simulink model "ssc_auto_ev_20b"  (R2020b)
settings: Solver=VariableStepAuto  StartTime=0.0  StopTime=200  RelTol=1e-3  AbsTol=1e-3
PreLoadFcn:
  | % Simulation parameters
  | dt = 0.01;
  | 
  | % Battery cell parameters
  | ssc_lithium_cell_1RC_ini
  | Nseries = 100;
  | Nparallel = 10;
  | 
  | % Motor parameters
  | max_torque = 220;
  | max_power = 80e3;
  | 
  | % Vehicle parameters
  | vehicle_mass = 4000;
  | wheel_radius = 0.35;
  | area = 5;
  | drag_coefficient = 0.25;
  | air_density = 1.225;
  | gravity = 9.81;
  | rolling_res_ratio = 0.015;
  | 
  | % Differential drive parameters
  | gear_ratio = 12;
  | 
  | % Simplified braking system parameters
  | force_max_pedal = 500;
  | braking_torque_to_pedal_force_ratio = -16;
  | 
  | % Vehicle controller parameters
  | hill_hold_max_speed = 0.5;
  | 
  | % Water properties for cooling circuit
  | load WaterProperties
  | 
  | % Input signals for Signal Editor block
  | load ssc_auto_ev_Inputs
values from neighbouring files (symbols this model uses):
  C1_LUT = [1913.6 4625.7 23306 10736 18036 12251 9022.9 12447 18872 40764 18721 33630 ... (21 elements, 7x3)]    [ssc_auto_ev_param.mat]
  Capacity_LUT = [28.0081 27.625 27.6392]    [ssc_auto_ev_param.mat]
  cell_Cp_heat = 810.5328    [ssc_auto_ev_param.mat]
  cell_mass = 1    [ssc_auto_ev_param.mat]
  Em_LUT = [3.4966 3.5519 3.6183 3.7066 3.9131 4.0748 4.1923 3.5057 3.566 3.6337 3.7127 3.9259 ... (21 elements, 7x3)]    [ssc_auto_ev_param.mat]
  Qe_init = 15.6845    [ssc_auto_ev_param.mat]
  R0_LUT = [0.0117 0.011 0.0114 0.0107 0.0107 0.0113 0.0116 0.0085 0.0085 0.0087 0.0082 0.0083 ... (21 elements, 7x3)]    [ssc_auto_ev_param.mat]
  R1_LUT = [0.0109 0.0069 0.0047 0.0034 0.0033 0.0033 0.0028 0.0029 0.0024 0.0026 0.0016 0.0023 ... (21 elements, 7x3)]    [ssc_auto_ev_param.mat]
  SOC_LUT = [0 0.1 0.25 0.5 0.75 0.9 1]    [ssc_auto_ev_param.mat]
  T_init = 293.15    [ssc_auto_ev_param.mat]
  Temperature_LUT = [278.15 293.15 313.15]    [ssc_auto_ev_param.mat]
undefined symbols (not defined in the file or in its folder): DiscIntNeverNeededParam, K, Lambda, tau, x0
libraries: fl_lib x656, nesl_utility x86, simulink x21, LiBatteryElements_lib x16, SignalEditorBlockLib x4, simulink_extras x4
(part 10 of 13)

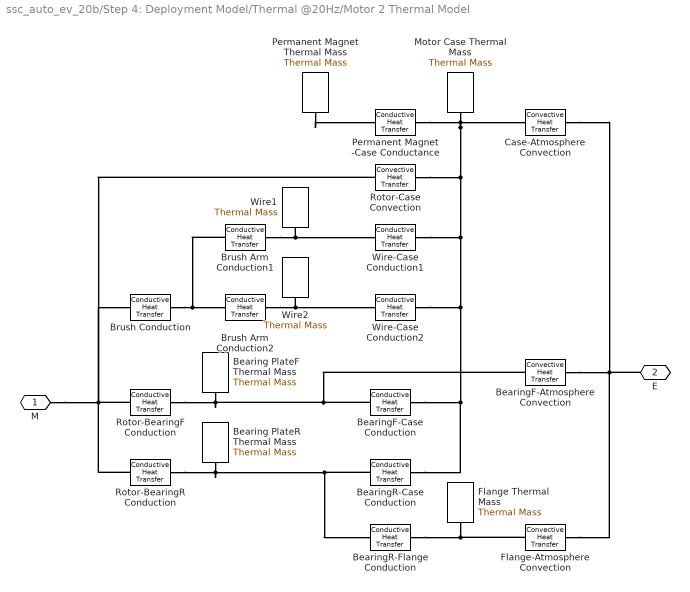
== system ssc_auto_ev_20b/Step 4: Deployment Model/Thermal @20Hz/Motor 2 Thermal Model ==
  Bearing PlateF Thermal Mass : fl_lib/Thermal/Thermal Elements/Thermal Mass  mass=0.6 kg  sp_heat=447 J/kg/K  T_specify=off  T_priority=High  T=300 K  T_nominal_specify=off  T_nominal_unit=K  T_nominal_value=1  Q_specify=off  Q_priority=None  Q=0 W  Q_nominal_specify=off  Q_nominal_unit=W  Q_nominal_value=1
      settings: SourceProductBaseCode=PW,SS,VE
  Bearing PlateR Thermal Mass : fl_lib/Thermal/Thermal Elements/Thermal Mass  mass=0.6 kg  sp_heat=447 J/kg/K  T_specify=off  T_priority=High  T=300 K  T_nominal_specify=off  T_nominal_unit=K  T_nominal_value=1  Q_specify=off  Q_priority=None  Q=0 W  Q_nominal_specify=off  Q_nominal_unit=W  Q_nominal_value=1
      settings: SourceProductBaseCode=PW,SS,VE
  BearingF-Atmosphere Convection : fl_lib/Thermal/Thermal Elements/Convective Heat Transfer  area=274.6 cm^2  heat_tr_coeff=123.5 W/(m^2 * K)  T_specify=off  T_priority=None  T=0 K  T_nominal_specify=off  T_nominal_unit=K  T_nominal_value=1  Q_specify=off  Q_priority=None  Q=0 W  Q_nominal_specify=off  Q_nominal_unit=W  Q_nominal_value=1
      settings: SourceProductBaseCode=PW,SS,VE
  BearingF-Case Conduction : fl_lib/Thermal/Thermal Elements/Conductive Heat Transfer  area=145 cm^2  thickness=18 cm  th_cond=80.2 W/(m*K)  T_specify=off  T_priority=None  T=0 K  T_nominal_specify=off  T_nominal_unit=K  T_nominal_value=1  Q_specify=off  Q_priority=None  Q=0 W  Q_nominal_specify=off  Q_nominal_unit=W  Q_nominal_value=1
      settings: SourceProductBaseCode=PW,SS,VE
  BearingR-Case Conduction : fl_lib/Thermal/Thermal Elements/Conductive Heat Transfer  area=145 cm^2  thickness=25 cm  th_cond=80.2 W/(m*K)  T_specify=off  T_priority=None  T=0 K  T_nominal_specify=off  T_nominal_unit=K  T_nominal_value=1  Q_specify=off  Q_priority=None  Q=0 W  Q_nominal_specify=off  Q_nominal_unit=W  Q_nominal_value=1
      settings: SourceProductBaseCode=PW,SS,VE
  BearingR-Flange Conduction : fl_lib/Thermal/Thermal Elements/Conductive Heat Transfer  area=34.5 cm^2  thickness=14 cm  th_cond=80.2 W/(m*K)  T_specify=off  T_priority=None  T=0 K  T_nominal_specify=off  T_nominal_unit=K  T_nominal_value=1  Q_specify=off  Q_priority=None  Q=0 W  Q_nominal_specify=off  Q_nominal_unit=W  Q_nominal_value=1
      settings: SourceProductBaseCode=PW,SS,VE
  Brush Conduction : fl_lib/Thermal/Thermal Elements/Conductive Heat Transfer  area=3*5 cm^2  thickness=4 cm  th_cond=1.7 W/(m*K)  T_specify=off  T_priority=None  T=0 K  T_nominal_specify=off  T_nominal_unit=K  T_nominal_value=1  Q_specify=off  Q_priority=None  Q=0 W  Q_nominal_specify=off  Q_nominal_unit=W  Q_nominal_value=1
      settings: SourceProductBaseCode=PW,SS,VE
  Brush Arm Conduction1 : fl_lib/Thermal/Thermal Elements/Conductive Heat Transfer  area=3*5 cm^2  thickness=4 cm  th_cond=1.7 W/(m*K)  T_specify=off  T_priority=None  T=0 K  T_nominal_specify=off  T_nominal_unit=K  T_nominal_value=1  Q_specify=off  Q_priority=None  Q=0 W  Q_nominal_specify=off  Q_nominal_unit=W  Q_nominal_value=1
      settings: SourceProductBaseCode=PW,SS,VE
  Brush Arm Conduction2 : fl_lib/Thermal/Thermal Elements/Conductive Heat Transfer  area=3*5 cm^2  thickness=4 cm  th_cond=1.7 W/(m*K)  T_specify=off  T_priority=None  T=0 K  T_nominal_specify=off  T_nominal_unit=K  T_nominal_value=1  Q_specify=off  Q_priority=None  Q=0 W  Q_nominal_specify=off  Q_nominal_unit=W  Q_nominal_value=1
      settings: SourceProductBaseCode=PW,SS,VE
  Case-Atmosphere Convection : fl_lib/Thermal/Thermal Elements/Convective Heat Transfer  area=4240 cm^2  heat_tr_coeff=26.8 W/(m^2 * K)  T_specify=off  T_priority=None  T=0 K  T_nominal_specify=off  T_nominal_unit=K  T_nominal_value=1  Q_specify=off  Q_priority=None  Q=0 W  Q_nominal_specify=off  Q_nominal_unit=W  Q_nominal_value=1
      settings: SourceProductBaseCode=PW,SS,VE
  Flange Thermal Mass : fl_lib/Thermal/Thermal Elements/Thermal Mass  mass=1.6 kg  sp_heat=447 J/kg/K  T_specify=off  T_priority=High  T=300 K  T_nominal_specify=off  T_nominal_unit=K  T_nominal_value=1  Q_specify=off  Q_priority=None  Q=0 W  Q_nominal_specify=off  Q_nominal_unit=W  Q_nominal_value=1
      settings: SourceProductBaseCode=PW,SS,VE
  Flange-Atmosphere Convection : fl_lib/Thermal/Thermal Elements/Convective Heat Transfer  area=324 cm^2  heat_tr_coeff=123.4 W/(m^2 * K)  T_specify=off  T_priority=None  T=0 K  T_nominal_specify=off  T_nominal_unit=K  T_nominal_value=1  Q_specify=off  Q_priority=None  Q=0 W  Q_nominal_specify=off  Q_nominal_unit=W  Q_nominal_value=1
      settings: SourceProductBaseCode=PW,SS,VE
  Motor Case Thermal Mass : fl_lib/Thermal/Thermal Elements/Thermal Mass  mass=3.8 kg  sp_heat=903 J/kg/K  T_specify=off  T_priority=High  T=300 K  T_nominal_specify=off  T_nominal_unit=K  T_nominal_value=1  Q_specify=off  Q_priority=None  Q=0 W  Q_nominal_specify=off  Q_nominal_unit=W  Q_nominal_value=1
      settings: SourceProductBaseCode=PW,SS,VE
  Permanent Magnet Thermal Mass : fl_lib/Thermal/Thermal Elements/Thermal Mass  mass=3.6 kg  sp_heat=447 J/kg/K  T_specify=off  T_priority=High  T=300 K  T_nominal_specify=off  T_nominal_unit=K  T_nominal_value=1  Q_specify=off  Q_priority=None  Q=0 W  Q_nominal_specify=off  Q_nominal_unit=W  Q_nominal_value=1
      settings: SourceProductBaseCode=PW,SS,VE
  Permanent Magnet -Case Conductance : fl_lib/Thermal/Thermal Elements/Conductive Heat Transfer  area=4350 cm^2  thickness=26 cm  th_cond=80.2 W/(m*K)  T_specify=off  T_priority=None  T=0 K  T_nominal_specify=off  T_nominal_unit=K  T_nominal_value=1  Q_specify=off  Q_priority=None  Q=0 W  Q_nominal_specify=off  Q_nominal_unit=W  Q_nominal_value=1
      settings: SourceProductBaseCode=PW,SS,VE
  Rotor-BearingF Conduction : fl_lib/Thermal/Thermal Elements/Conductive Heat Transfer  area=26.4 cm^2  thickness=2.5 cm  th_cond=80.2 W/(m*K)  T_specify=off  T_priority=None  T=0 K  T_nominal_specify=off  T_nominal_unit=K  T_nominal_value=1  Q_specify=off  Q_priority=None  Q=0 W  Q_nominal_specify=off  Q_nominal_unit=W  Q_nominal_value=1
      settings: SourceProductBaseCode=PW,SS,VE
  Rotor-BearingR Conduction : fl_lib/Thermal/Thermal Elements/Conductive Heat Transfer  area=26.4 cm^2  thickness=2.5 cm  th_cond=80.2 W/(m*K)  T_specify=off  T_priority=None  T=0 K  T_nominal_specify=off  T_nominal_unit=K  T_nominal_value=1  Q_specify=off  Q_priority=None  Q=0 W  Q_nominal_specify=off  Q_nominal_unit=W  Q_nominal_value=1
      settings: SourceProductBaseCode=PW,SS,VE
  Rotor-Case Convection : fl_lib/Thermal/Thermal Elements/Convective Heat Transfer  area=1240 cm^2  heat_tr_coeff=210 W/(m^2 * K)  T_specify=off  T_priority=None  T=0 K  T_nominal_specify=off  T_nominal_unit=K  T_nominal_value=1  Q_specify=off  Q_priority=None  Q=0 W  Q_nominal_specify=off  Q_nominal_unit=W  Q_nominal_value=1
      settings: SourceProductBaseCode=PW,SS,VE
  Wire-Case Conduction1 : fl_lib/Thermal/Thermal Elements/Conductive Heat Transfer  area=1 cm^2  thickness=0.2 cm  th_cond=4 W/(m*K)  T_specify=off  T_priority=None  T=0 K  T_nominal_specify=off  T_nominal_unit=K  T_nominal_value=1  Q_specify=off  Q_priority=None  Q=0 W  Q_nominal_specify=off  Q_nominal_unit=W  Q_nominal_value=1
      settings: SourceProductBaseCode=PW,SS,VE
  Wire-Case Conduction2 : fl_lib/Thermal/Thermal Elements/Conductive Heat Transfer  area=1 cm^2  thickness=0.2 cm  th_cond=4 W/(m*K)  T_specify=off  T_priority=None  T=0 K  T_nominal_specify=off  T_nominal_unit=K  T_nominal_value=1  Q_specify=off  Q_priority=None  Q=0 W  Q_nominal_specify=off  Q_nominal_unit=W  Q_nominal_value=1
      settings: SourceProductBaseCode=PW,SS,VE
  Wire1 : fl_lib/Thermal/Thermal Elements/Thermal Mass  mass=0.05 kg  sp_heat=385 J/kg/K  T_specify=off  T_priority=High  T=300 K  T_nominal_specify=off  T_nominal_unit=K  T_nominal_value=1  Q_specify=off  Q_priority=None  Q=0 W  Q_nominal_specify=off  Q_nominal_unit=W  Q_nominal_value=1
      settings: SourceProductBaseCode=PW,SS,VE
  Wire2 : fl_lib/Thermal/Thermal Elements/Thermal Mass  mass=0.05 kg  sp_heat=385 J/kg/K  T_specify=off  T_priority=High  T=300 K  T_nominal_specify=off  T_nominal_unit=K  T_nominal_value=1  Q_specify=off  Q_priority=None  Q=0 W  Q_nominal_specify=off  Q_nominal_unit=W  Q_nominal_value=1
      settings: SourceProductBaseCode=PW,SS,VE
  M : PMIOPort  Side=Right
  E : PMIOPort  Port=2  Side=Left
  connections:
  Flange-Atmosphere Convection/RConn1 -- E/RConn1 -- BearingF-Atmosphere Convection/RConn1 -- Case-Atmosphere Convection/RConn1
  Motor Case Thermal Mass/LConn1 -- Case-Atmosphere Convection/LConn1 -- Permanent Magnet -Case Conductance/RConn1 -- Wire-Case Conduction1/RConn1 -- Wire-Case Conduction2/RConn1 -- BearingF-Case Conduction/RConn1 -- BearingR-Case Conduction/RConn1 -- Rotor-Case Convection/RConn1
  Rotor-BearingR Conduction/RConn1 -- Bearing PlateR Thermal Mass/LConn1 -- BearingR-Flange Conduction/LConn1 -- BearingR-Case Conduction/LConn1
  Flange-Atmosphere Convection/LConn1 -- BearingR-Flange Conduction/RConn1 -- Flange Thermal Mass/LConn1
  BearingF-Case Conduction/LConn1 -- BearingF-Atmosphere Convection/LConn1 -- Rotor-BearingF Conduction/RConn1 -- Bearing PlateF Thermal Mass/LConn1
  M/RConn1 -- Rotor-Case Convection/LConn1 -- Brush Conduction/LConn1 -- Rotor-BearingR Conduction/LConn1 -- Rotor-BearingF Conduction/LConn1
  Permanent Magnet Thermal Mass/LConn1 -- Permanent Magnet -Case Conductance/LConn1
  Brush Conduction/RConn1 -- Brush Arm Conduction1/LConn1 -- Brush Arm Conduction2/LConn1
  Brush Arm Conduction1/RConn1 -- Wire-Case Conduction1/LConn1 -- Wire1/LConn1
  Brush Arm Conduction2/RConn1 -- Wire-Case Conduction2/LConn1 -- Wire2/LConn1

== system ssc_auto_ev_20b/Step 4: Deployment Model/Thermal @20Hz/Port 2 Interface ==
  temperature : Inport
  Controlled Temperature Source : fl_lib/Thermal/Thermal Sources/Controlled Temperature Source
      settings: SourceProductBaseCode=PW,SS,VE
  Heat Flow Rate Sensor : fl_lib/Thermal/Thermal Sensors/Heat Flow Rate Sensor
      settings: SourceProductBaseCode=PW,SS,VE
  T2 : nesl_utility/Simulink-PS Converter  PhysicalDomain=network_engine_domain  SubClassName=ps_input  LeftPortType=input  RightPortType=output  PseudoPeriodic=off  Frequencies=[]  NoiseDistribution=none  NoiseParameters=[]  Unit=K  AffineConversion=off  FilteringAndDerivatives=provide  SimscapeFilterOrder=1  InputFilterTimeConstant=0.001  UdotUserProvided=0
      settings: SourceProductBaseCode=SS,PW,VE
  Thermal Reference : fl_lib/Thermal/Thermal Elements/Thermal Reference
      settings: SourceProductBaseCode=PW,SS,VE
  q2 : nesl_utility/PS-Simulink Converter  PhysicalDomain=network_engine_domain  SubClassName=ps_output  LeftPortType=input  RightPortType=output  PseudoPeriodic=off  Frequencies=[]  Unit=W  AffineConversion=off
      settings: SourceProductBaseCode=SS,PW,VE
  2 : PMIOPort  Side=Right
  heat flow : Outport
  wires:
  q2/1 -> heat flow/1
  temperature/1 -> T2/1
  connections:
  Heat Flow Rate Sensor/RConn2 -- Controlled Temperature Source/LConn1
  Thermal Reference/LConn1 -- Controlled Temperature Source/RConn2
  Heat Flow Rate Sensor/LConn1 -- 2/RConn1
  T2/RConn1 -- Controlled Temperature Source/RConn1
  q2/LConn1 -- Heat Flow Rate Sensor/RConn1

== system ssc_auto_ev_20b/Step 4: Deployment Model/Thermal @20Hz/Port 2 Interface1 ==
  temperature : Inport
  Controlled Temperature Source : fl_lib/Thermal/Thermal Sources/Controlled Temperature Source
      settings: SourceProductBaseCode=PW,SS,VE
  Heat Flow Rate Sensor : fl_lib/Thermal/Thermal Sensors/Heat Flow Rate Sensor
      settings: SourceProductBaseCode=PW,SS,VE
  T2 : nesl_utility/Simulink-PS Converter  PhysicalDomain=network_engine_domain  SubClassName=ps_input  LeftPortType=input  RightPortType=output  PseudoPeriodic=off  Frequencies=[]  NoiseDistribution=none  NoiseParameters=[]  Unit=K  AffineConversion=off  FilteringAndDerivatives=provide  SimscapeFilterOrder=1  InputFilterTimeConstant=0.001  UdotUserProvided=0
      settings: SourceProductBaseCode=SS,PW,VE
  Thermal Reference : fl_lib/Thermal/Thermal Elements/Thermal Reference
      settings: SourceProductBaseCode=PW,SS,VE
  q2 : nesl_utility/PS-Simulink Converter  PhysicalDomain=network_engine_domain  SubClassName=ps_output  LeftPortType=input  RightPortType=output  PseudoPeriodic=off  Frequencies=[]  Unit=W  AffineConversion=off
      settings: SourceProductBaseCode=SS,PW,VE
  2 : PMIOPort  Side=Right
  heat flow : Outport
  wires:
  q2/1 -> heat flow/1
  temperature/1 -> T2/1
  connections:
  Heat Flow Rate Sensor/RConn2 -- Controlled Temperature Source/LConn1
  Thermal Reference/LConn1 -- Controlled Temperature Source/RConn2
  Heat Flow Rate Sensor/LConn1 -- 2/RConn1
  T2/RConn1 -- Controlled Temperature Source/RConn1
  q2/LConn1 -- Heat Flow Rate Sensor/RConn1

== system ssc_auto_ev_20b/Step 4: Deployment Model/Thermal @20Hz/Port 2 Interface2 ==
  temperature : Inport
  Controlled Temperature Source : fl_lib/Thermal/Thermal Sources/Controlled Temperature Source
      settings: SourceProductBaseCode=PW,SS,VE
  Heat Flow Rate Sensor : fl_lib/Thermal/Thermal Sensors/Heat Flow Rate Sensor
      settings: SourceProductBaseCode=PW,SS,VE
  T2 : nesl_utility/Simulink-PS Converter  PhysicalDomain=network_engine_domain  SubClassName=ps_input  LeftPortType=input  RightPortType=output  PseudoPeriodic=off  Frequencies=[]  NoiseDistribution=none  NoiseParameters=[]  Unit=K  AffineConversion=off  FilteringAndDerivatives=provide  SimscapeFilterOrder=1  InputFilterTimeConstant=0.001  UdotUserProvided=0
      settings: SourceProductBaseCode=SS,PW,VE
  Thermal Reference : fl_lib/Thermal/Thermal Elements/Thermal Reference
      settings: SourceProductBaseCode=PW,SS,VE
  q2 : nesl_utility/PS-Simulink Converter  PhysicalDomain=network_engine_domain  SubClassName=ps_output  LeftPortType=input  RightPortType=output  PseudoPeriodic=off  Frequencies=[]  Unit=W  AffineConversion=off
      settings: SourceProductBaseCode=SS,PW,VE
  2 : PMIOPort  Side=Right
  heat flow : Outport
  wires:
  temperature/1 -> T2/1
  q2/1 -> heat flow/1
  connections:
  q2/LConn1 -- Heat Flow Rate Sensor/RConn1
  T2/RConn1 -- Controlled Temperature Source/RConn1
  Heat Flow Rate Sensor/LConn1 -- 2/RConn1
  Thermal Reference/LConn1 -- Controlled Temperature Source/RConn2
  Heat Flow Rate Sensor/RConn2 -- Controlled Temperature Source/LConn1

== system ssc_auto_ev_20b/Step 4: Deployment Model/Vehicle and drive @100Hz/Motor Drive ==
  iRef : Inport
  DC Motor1 : Subsystem  Tag=PublishSubsystem
      mask Display:
      | % Circle, in/out, and 'M'
      | image('ssc_dcmotor_maskicon.png');
      | 
      | % % Circle
      | % plot(sin(0:0.1:2.2*pi)*0.9,cos(0:0.1:2.2*pi)*0.9);
      | %
      | % % In/out
      | % plot([-1.3 -0.9],[0 0]);
      | % plot([1.3 0.9],[0 0]);
      | %
      | % % 'M'
      | % plot([0.5 0.5],[-0.5 0.5]);
      | % plot([-0.5 -0.5],[-0.5 0.5]);
      | % plot([0.5 0],[0.5 -0.5]);
      | % plot([-0.5 0],[0.5 -0.5]);
      | 
      | % Plot points to set plot range
      | color('white');plot(1.5,1.5);plot(-1.5,-1.5)
      | color('black');
      | 
      | port_label('RConn',1,'R');
      | port_label('RConn',2,'C');
      | port_label('LConn',1,'V+');
      | port_label('LConn',2,'V-');
  DC Motor2 : Subsystem  Tag=PublishSubsystem
      mask Display:
      | % Circle, in/out, and 'M'
      | image('ssc_dcmotor_maskicon.png');
      | 
      | % % Circle
      | % plot(sin(0:0.1:2.2*pi)*0.9,cos(0:0.1:2.2*pi)*0.9);
      | %
      | % % In/out
      | % plot([-1.3 -0.9],[0 0]);
      | % plot([1.3 0.9],[0 0]);
      | %
      | % % 'M'
      | % plot([0.5 0.5],[-0.5 0.5]);
      | % plot([-0.5 -0.5],[-0.5 0.5]);
      | % plot([0.5 0],[0.5 -0.5]);
      | % plot([-0.5 0],[0.5 -0.5]);
      | 
      | % Plot points to set plot range
      | color('white');plot(1.5,1.5);plot(-1.5,-1.5)
      | color('black');
      | 
      | port_label('RConn',1,'R');
      | port_label('RConn',2,'C');
      | port_label('LConn',1,'V+');
      | port_label('LConn',2,'V-');
  Ideal Rotational Motion Sensor : fl_lib/Mechanical/Mechanical Sensors/Ideal Rotational Motion Sensor  wrap_angle=simscape.enum.onoff.off  offset=0 rad
      settings: SourceProductBaseCode=PW,SS,VE
  MRRef : fl_lib/Mechanical/Rotational Elements/Mechanical Rotational Reference
      settings: SourceProductBaseCode=PW,SS,VE
  MRRef1 : fl_lib/Mechanical/Rotational Elements/Mechanical Rotational Reference
      settings: SourceProductBaseCode=PW,SS,VE
  MRRef2 : fl_lib/Mechanical/Rotational Elements/Mechanical Rotational Reference
      settings: SourceProductBaseCode=PW,SS,VE
  Motor Torque Controller 1 (System-Level Representation) : Subsystem
      settings: PortSchema="{\"entries\":[{\"content\":{\"sides\":[{\"content\":{\"connectorIds\":[\"LConn1\",\"LConn2\"]},\"type\":\"ConnectorPlacement.EquallySpacedRectSide\",\"uuid\":\"fa610323-4e51-4b68-84d8-5520af174050\"},{\"content\":{\"connectorIds\":[\"RConn1\",\"RConn2\"],\"side\":\"RIGHT\"},\"type\":\"ConnectorPlacement.EquallySpacedRectSide\",\"uuid\":\"4363b90b-a4e0-4b49-9dec-cc6d130d9345\"},{\"content\":{\"connectorIds\":[\"LConn3\"],\"side\":\"TOP\"},\"type\":\"ConnectorPlacement.EquallySpacedRectSide\",\"uuid\":\"1b5285b6-bf42-4633-bccd-78a8c0464c36\"}]},\"type\":\"ConnectorPlacement.EquallySpacedConnector\",\"uuid\":\"5522e717-4ae9-420d-ac3d-a671d244aac1\"}],\"packageUris\":[\"http://schema.mathworks.com/mf0/Connector/R2020b\"],\"version\":\"1.0\"}"
  Motor Torque Controller 1 (System-Level Representation)1 : Subsystem
      settings: PortSchema="{\"entries\":[{\"content\":{\"sides\":[{\"content\":{\"connectorIds\":[\"LConn1\",\"LConn2\"]},\"type\":\"ConnectorPlacement.EquallySpacedRectSide\",\"uuid\":\"fa610323-4e51-4b68-84d8-5520af174050\"},{\"content\":{\"connectorIds\":[\"RConn1\",\"RConn2\"],\"side\":\"RIGHT\"},\"type\":\"ConnectorPlacement.EquallySpacedRectSide\",\"uuid\":\"4363b90b-a4e0-4b49-9dec-cc6d130d9345\"},{\"content\":{\"connectorIds\":[\"LConn3\"],\"side\":\"TOP\"},\"type\":\"ConnectorPlacement.EquallySpacedRectSide\",\"uuid\":\"1b5285b6-bf42-4633-bccd-78a8c0464c36\"}]},\"type\":\"ConnectorPlacement.EquallySpacedConnector\",\"uuid\":\"5522e717-4ae9-420d-ac3d-a671d244aac1\"}],\"packageUris\":[\"http://schema.mathworks.com/mf0/Connector/R2020b\"],\"version\":\"1.0\"}"
  Sensing wMotor : Subsystem
      mask Display: disp('w');
  Simulink-PS G1 : nesl_utility/Simulink-PS Converter  PhysicalDomain=network_engine_domain  SubClassName=ps_input  LeftPortType=input  RightPortType=output  PseudoPeriodic=off  Frequencies=[]  NoiseDistribution=none  NoiseParameters=[]  Unit=A  AffineConversion=off  FilteringAndDerivatives=zero  SimscapeFilterOrder=1  InputFilterTimeConstant=1e-6  UdotUserProvided=1
      settings: SourceProductBaseCode=SS,PW,VE
  Winding-Iron Conductance/1 : fl_lib/Thermal/Thermal Elements/Conductive Heat Transfer  area=250 cm^2  thickness=0.2 cm  th_cond=360 W/(m*K)  T_specify=off  T_priority=None  T=0 K  T_nominal_specify=off  T_nominal_unit=K  T_nominal_value=1  Q_specify=off  Q_priority=None  Q=0 W  Q_nominal_specify=off  Q_nominal_unit=W  Q_nominal_value=1
      settings: SourceProductBaseCode=PW,SS,VE
  Winding-Iron Conductance/2 : fl_lib/Thermal/Thermal Elements/Conductive Heat Transfer  area=250 cm^2  thickness=0.2 cm  th_cond=360 W/(m*K)  T_specify=off  T_priority=None  T=0 K  T_nominal_specify=off  T_nominal_unit=K  T_nominal_value=1  Q_specify=off  Q_priority=None  Q=0 W  Q_nominal_specify=off  Q_nominal_unit=W  Q_nominal_value=1
      settings: SourceProductBaseCode=PW,SS,VE
  + : PMIOPort  Side=Left
  - : PMIOPort  Port=2  Side=Left
  R : PMIOPort  Port=3  Side=Right
  M1 : PMIOPort  Port=4  Side=Left
  M2 : PMIOPort  Port=5  Side=Left
  w : Outport  VectorParamsAs1DForOutWhenUnconnected=off
  wires:
  iRef/1 -> Simulink-PS G1/1
  Sensing wMotor/1(SL) -> w/1
  connections:
  M2/RConn1 -- Winding-Iron Conductance/2/LConn1
  M1/RConn1 -- Winding-Iron Conductance/1/LConn1
  Winding-Iron Conductance/2/RConn1 -- DC Motor2/LConn3
  Winding-Iron Conductance/1/RConn1 -- DC Motor1/LConn3
  DC Motor2/LConn2 -- Motor Torque Controller 1 (System-Level Representation)1/LConn2
  DC Motor2/LConn1 -- Motor Torque Controller 1 (System-Level Representation)1/LConn1
  DC Motor2/RConn2 -- MRRef2/LConn1
  Motor Torque Controller 1 (System-Level Representation)1/LConn3 -- Motor Torque Controller 1 (System-Level Representation)/LConn3 -- Simulink-PS G1/RConn1
  DC Motor1/LConn2 -- Motor Torque Controller 1 (System-Level Representation)/LConn2
  Motor Torque Controller 1 (System-Level Representation)/RConn2 -- Motor Torque Controller 1 (System-Level Representation)1/RConn2 -- -/RConn1
  Motor Torque Controller 1 (System-Level Representation)/RConn1 -- Motor Torque Controller 1 (System-Level Representation)1/RConn1 -- +/RConn1
  Motor Torque Controller 1 (System-Level Representation)/LConn1 -- DC Motor1/LConn1
  MRRef1/LConn1 -- Ideal Rotational Motion Sensor/RConn1
  DC Motor1/RConn2 -- MRRef/LConn1
  R/RConn1 -- Ideal Rotational Motion Sensor/LConn1 -- DC Motor2/RConn1 -- DC Motor1/RConn1
  Ideal Rotational Motion Sensor/RConn2 -- Sensing wMotor/LConn1

== system ssc_auto_ev_20b/Step 4: Deployment Model/Vehicle and drive @100Hz/Port 1 Interface1 ==
  heat flow : Inport
  Controlled Temperature Source : fl_lib/Thermal/Thermal Sources/Controlled Temperature Source
      settings: SourceProductBaseCode=PW,SS,VE
  Heat Flow Rate Sensor : fl_lib/Thermal/Thermal Sensors/Heat Flow Rate Sensor
      settings: SourceProductBaseCode=PW,SS,VE
  Interface : Subsystem  Variant=on  VariantControlMode=label  VariantControl=Variant1  LabelModeActiveChoice=Discrete
      settings: PortSchema="{\"entries\":[{\"content\":{\"sides\":[{\"content\":{\"connectorIds\":[\"In1\",\"Out2\"]},\"type\":\"ConnectorPlacement.EquallySpacedRectSide\",\"uuid\":\"aa56821c-7799-44e3-b228-553c5b43a68d\"},{\"content\":{\"connectorIds\":[\"In2\",\"Out1\"],\"side\":\"RIGHT\"},\"type\":\"ConnectorPlacement.EquallySpacedRectSide\",\"uuid\":\"8658dee5-55e2-4f33-bdec-e6600ce27fc1\"},{\"content\":{\"connectorIds\":[],\"side\":\"TOP\"},\"type\":\"ConnectorPlacement.EquallySpacedRectSide\",\"uuid\":\"2effe9c6-8e61-4f0c-a39b-329d9ffc707d\"}]},\"type\":\"ConnectorPlacement.EquallySpacedConnector\",\"uuid\":\"c8fc8444-dfc7-49a5-9550-b957635f7d8f\"}],\"packageUris\":[\"http://schema.mathworks.com/mf0/Connector/R2020b\"],\"version\":\"1.0\"}"
  T1 : nesl_utility/Simulink-PS Converter  PhysicalDomain=network_engine_domain  SubClassName=ps_input  LeftPortType=input  RightPortType=output  PseudoPeriodic=off  Frequencies=[]  NoiseDistribution=none  NoiseParameters=[]  Unit=K  AffineConversion=off  FilteringAndDerivatives=provide  SimscapeFilterOrder=1  InputFilterTimeConstant=0.001  UdotUserProvided=0
      settings: SourceProductBaseCode=SS,PW,VE
  Thermal Reference : fl_lib/Thermal/Thermal Elements/Thermal Reference
      settings: SourceProductBaseCode=PW,SS,VE
  q1 : nesl_utility/PS-Simulink Converter  PhysicalDomain=network_engine_domain  SubClassName=ps_output  LeftPortType=input  RightPortType=output  PseudoPeriodic=off  Frequencies=[]  Unit=W  AffineConversion=off
      settings: SourceProductBaseCode=SS,PW,VE
  1 : PMIOPort  Side=Left
  temperature : Outport
  wires:
  Interface/1(across2) -> temperature/1
  q1/1 -> Interface/1(through1)
  heat flow/1 -> Interface/2(through2)
  Interface/2(across1) -> T1/1
  connections:
  Heat Flow Rate Sensor/RConn2 -- Controlled Temperature Source/LConn1
  Heat Flow Rate Sensor/LConn1 -- 1/RConn1
  q1/LConn1 -- Heat Flow Rate Sensor/RConn1
  Thermal Reference/LConn1 -- Controlled Temperature Source/RConn2
  Controlled Temperature Source/RConn1 -- T1/RConn1

== system ssc_auto_ev_20b/Step 4: Deployment Model/Vehicle and drive @100Hz/Port 1 Interface2 ==
  heat flow : Inport
  Controlled Temperature Source : fl_lib/Thermal/Thermal Sources/Controlled Temperature Source
      settings: SourceProductBaseCode=PW,SS,VE
  Heat Flow Rate Sensor : fl_lib/Thermal/Thermal Sensors/Heat Flow Rate Sensor
      settings: SourceProductBaseCode=PW,SS,VE
  Interface : Subsystem  Variant=on  VariantControlMode=label  VariantControl=Variant1  LabelModeActiveChoice=Discrete
      settings: PortSchema="{\"entries\":[{\"content\":{\"sides\":[{\"content\":{\"connectorIds\":[\"In1\",\"Out2\"]},\"type\":\"ConnectorPlacement.EquallySpacedRectSide\",\"uuid\":\"aa56821c-7799-44e3-b228-553c5b43a68d\"},{\"content\":{\"connectorIds\":[\"In2\",\"Out1\"],\"side\":\"RIGHT\"},\"type\":\"ConnectorPlacement.EquallySpacedRectSide\",\"uuid\":\"8658dee5-55e2-4f33-bdec-e6600ce27fc1\"},{\"content\":{\"connectorIds\":[],\"side\":\"TOP\"},\"type\":\"ConnectorPlacement.EquallySpacedRectSide\",\"uuid\":\"2effe9c6-8e61-4f0c-a39b-329d9ffc707d\"}]},\"type\":\"ConnectorPlacement.EquallySpacedConnector\",\"uuid\":\"c8fc8444-dfc7-49a5-9550-b957635f7d8f\"}],\"packageUris\":[\"http://schema.mathworks.com/mf0/Connector/R2020b\"],\"version\":\"1.0\"}"
  T1 : nesl_utility/Simulink-PS Converter  PhysicalDomain=network_engine_domain  SubClassName=ps_input  LeftPortType=input  RightPortType=output  PseudoPeriodic=off  Frequencies=[]  NoiseDistribution=none  NoiseParameters=[]  Unit=K  AffineConversion=off  FilteringAndDerivatives=provide  SimscapeFilterOrder=1  InputFilterTimeConstant=0.001  UdotUserProvided=0
      settings: SourceProductBaseCode=SS,PW,VE
  Thermal Reference : fl_lib/Thermal/Thermal Elements/Thermal Reference
      settings: SourceProductBaseCode=PW,SS,VE
  q1 : nesl_utility/PS-Simulink Converter  PhysicalDomain=network_engine_domain  SubClassName=ps_output  LeftPortType=input  RightPortType=output  PseudoPeriodic=off  Frequencies=[]  Unit=W  AffineConversion=off
      settings: SourceProductBaseCode=SS,PW,VE
  1 : PMIOPort  Side=Left
  temperature : Outport
  wires:
  Interface/2(across1) -> T1/1
  heat flow/1 -> Interface/2(through2)
  q1/1 -> Interface/1(through1)
  Interface/1(across2) -> temperature/1
  connections:
  Controlled Temperature Source/RConn1 -- T1/RConn1
  Thermal Reference/LConn1 -- Controlled Temperature Source/RConn2
  q1/LConn1 -- Heat Flow Rate Sensor/RConn1
  Heat Flow Rate Sensor/LConn1 -- 1/RConn1
  Heat Flow Rate Sensor/RConn2 -- Controlled Temperature Source/LConn1

== system ssc_auto_ev_20b/Step 4: Deployment Model/Vehicle and drive @100Hz/Port 1 Interface3 ==
  voltage : Inport
  Controlled Voltage Source : fl_lib/Electrical/Electrical Sources/Controlled Voltage Source
      settings: SourceProductBaseCode=PW,SS,VE
  Current Sensor : fl_lib/Electrical/Electrical Sensors/Current Sensor
      settings: SourceProductBaseCode=PW,SS,VE
  Electrical Reference : fl_lib/Electrical/Electrical Elements/Electrical Reference
      settings: SourceProductBaseCode=PW,SS,VE
  Interface : Subsystem  Variant=on  VariantControlMode=label  VariantControl=Variant1  LabelModeActiveChoice=Discrete
      settings: PortSchema="{\"entries\":[{\"content\":{\"sides\":[{\"content\":{\"connectorIds\":[\"In1\",\"Out2\"]},\"type\":\"ConnectorPlacement.EquallySpacedRectSide\",\"uuid\":\"aa56821c-7799-44e3-b228-553c5b43a68d\"},{\"content\":{\"connectorIds\":[\"In2\",\"Out1\"],\"side\":\"RIGHT\"},\"type\":\"ConnectorPlacement.EquallySpacedRectSide\",\"uuid\":\"8658dee5-55e2-4f33-bdec-e6600ce27fc1\"},{\"content\":{\"connectorIds\":[],\"side\":\"TOP\"},\"type\":\"ConnectorPlacement.EquallySpacedRectSide\",\"uuid\":\"2effe9c6-8e61-4f0c-a39b-329d9ffc707d\"}]},\"type\":\"ConnectorPlacement.EquallySpacedConnector\",\"uuid\":\"c8fc8444-dfc7-49a5-9550-b957635f7d8f\"}],\"packageUris\":[\"http://schema.mathworks.com/mf0/Connector/R2020b\"],\"version\":\"1.0\"}"
  Ip : nesl_utility/PS-Simulink Converter  PhysicalDomain=network_engine_domain  SubClassName=ps_output  LeftPortType=input  RightPortType=output  PseudoPeriodic=off  Frequencies=[]  Unit=A  AffineConversion=off
      settings: SourceProductBaseCode=SS,PW,VE
  Vp : nesl_utility/Simulink-PS Converter  PhysicalDomain=network_engine_domain  SubClassName=ps_input  LeftPortType=input  RightPortType=output  PseudoPeriodic=off  Frequencies=[]  NoiseDistribution=none  NoiseParameters=[]  Unit=V  AffineConversion=off  FilteringAndDerivatives=zero  SimscapeFilterOrder=1  InputFilterTimeConstant=0.001  UdotUserProvided=1
      settings: SourceProductBaseCode=SS,PW,VE
  1 : PMIOPort  Side=Left
  current : Outport
  wires:
  voltage/1 -> Interface/2(across2)
  Interface/2(across1) -> Vp/1
  Ip/1 -> Interface/1(through1)
  Interface/1(through2) -> current/1
  connections:
  Vp/RConn1 -- Controlled Voltage Source/RConn1
  1/RConn1 -- Current Sensor/LConn1
  Current Sensor/RConn2 -- Controlled Voltage Source/LConn1
  Current Sensor/RConn1 -- Ip/LConn1
  Electrical Reference/LConn1 -- Controlled Voltage Source/RConn2

== system ssc_auto_ev_20b/Step 4: Deployment Model/Vehicle and drive @100Hz/Vehicle Dynamics ==
  Test data : Inport
  Brake Torque : Subsystem
  Bus Selector : BusSelector  OutputSignals=Incline,Wind speed,Brake pedal
  Drag and Gravity : Subsystem
  Final Drive Ratio : fl_lib/Mechanical/Mechanisms/Gear Box  ratio=gear_ratio  t_in_specify=off  t_in_priority=High  t_in=0 N*m  t_in_nominal_specify=off  t_in_nominal_unit=N*m  t_in_nominal_value=1  t_out_specify=off  t_out_priority=High  t_out=0 N*m  t_out_nominal_specify=off  t_out_nominal_unit=N*m  t_out_nominal_value=1
      settings: SourceProductBaseCode=PW,SS,VE
  Force Source : fl_lib/Mechanical/Mechanical Sources/Ideal Force Source
      settings: SourceProductBaseCode=PW,SS,VE
  MTRef : fl_lib/Mechanical/Translational Elements/Mechanical Translational Reference
      settings: SourceProductBaseCode=PW,SS,VE
  PS Subtract : fl_lib/Physical Signals/Functions/PS Subtract
      settings: SourceProductBaseCode=PW,SS,VE
  Sensing Speed : Subsystem
      mask Display: disp('v')
  Vehicle Mass : fl_lib/Mechanical/Translational Elements/Mass  mass=vehicle_mass kg  num_ports=foundation.enum.numPorts2.one  v_specify=off  v_priority=High  v=0 m/s  v_nominal_specify=off  v_nominal_unit=m/s  v_nominal_value=1  f_specify=off  f_priority=High  f=0 N  f_nominal_specify=off  f_nominal_unit=N  f_nominal_value=1
      settings: SourceProductBaseCode=PW,SS,VE
  Wheel and Axle : fl_lib/Mechanical/Mechanisms/Wheel and Axle  R=wheel_radius m  or=1  t_specify=off  t_priority=High  t=0 N*m  t_nominal_specify=off  t_nominal_unit=N*m  t_nominal_value=1  f_specify=off  f_priority=High  f=0 N  f_nominal_specify=off  f_nominal_unit=N  f_nominal_value=1
      settings: SourceProductBaseCode=PW,SS,VE
  R : PMIOPort  Side=Left
  wires:
  Test data/1 -> Bus Selector/1
  Bus Selector/3 -> Brake Torque/1(Pedal)  "<Brake pedal>"
  Bus Selector/1 -> Drag and Gravity/1(beta)  "<Incline>"
  Bus Selector/2 -> Drag and Gravity/2(vW)  "<Wind speed>"
  connections:
  R/RConn1 -- Final Drive Ratio/LConn1
  Force Source/RConn2 -- MTRef/LConn1
  Brake Torque/RConn1 -- Final Drive Ratio/RConn1 -- Wheel and Axle/LConn1
  PS Subtract/RConn1 -- Force Source/RConn1
  Drag and Gravity/LConn3 -- PS Subtract/LConn1
  Drag and Gravity/LConn2 -- PS Subtract/LConn2
  Wheel and Axle/RConn1 -- Sensing Speed/LConn1 -- Force Source/LConn1 -- Vehicle Mass/LConn1
  Drag and Gravity/LConn1 -- Sensing Speed/RConn1

== system ssc_auto_ev_20b/Vehicle Dynamics/Brake Torque/Smooth Sign ==
  1 : fl_lib/Physical Signals/Sources/PS Constant  constant=1
      settings: SourceProductBaseCode=PW,SS,VE
  2 : fl_lib/Physical Signals/Functions/PS Gain  gain=2 1/(rad/s)
      settings: SourceProductBaseCode=PW,SS,VE
  PS Add : fl_lib/Physical Signals/Functions/PS Add
      settings: SourceProductBaseCode=PW,SS,VE
  PS Subtract : fl_lib/Physical Signals/Functions/PS Subtract
      settings: SourceProductBaseCode=PW,SS,VE
  exp(2x) : fl_lib/Physical Signals/Functions/PS Math Function  fcn_choice=foundation.enum.math_function.exp
      settings: SourceProductBaseCode=PW,SS,VE
  tanh(x) : fl_lib/Physical Signals/Functions/PS Divide
      settings: SourceProductBaseCode=PW,SS,VE
  x : PMIOPort  Side=Left
  y : PMIOPort  Port=2  Side=Right
  connections:
  1/RConn1 -- PS Subtract/LConn2 -- PS Add/LConn1
  exp(2x)/LConn1 -- 2/RConn1
  exp(2x)/RConn1 -- PS Subtract/LConn1 -- PS Add/LConn2
  tanh(x)/LConn2 -- PS Add/RConn1
  tanh(x)/LConn1 -- PS Subtract/RConn1
  2/LConn1 -- x/RConn1
  tanh(x)/RConn1 -- y/RConn1

== system ssc_auto_ev_20b/Vehicle Control/Cruise Control/Capture speed ==
  In1 : Inport
  Trigger : TriggerPort  VariantControl=Variant
  Out1 : Outport  VectorParamsAs1DForOutWhenUnconnected=off
  wires:
  In1/1 -> Out1/1

== system ssc_auto_ev_20b/Vehicle Control/Cruise Control/Speed Controller ==
  wRef : Inport
  wMeas : Inport  Port=2
  Add : Sum  Inputs=|+-
  Add1 : Sum
  Discrete-Time Integrator : DiscreteIntegrator  gainval=Ki  SampleTime=ts  LimitOutput=on  UpperSaturationLimit=trqMax  LowerSaturationLimit=-trqMax  ICPrevOutput=DiscIntNeverNeededParam  ICPrevScaledInput=DiscIntNeverNeededParam
  Kp : Gain  Gain=Kp
  trqRef : Outport  VectorParamsAs1DForOutWhenUnconnected=off
  wires:
  Add/1 -> Discrete-Time Integrator/1, Kp/1
  Add1/1 -> trqRef/1
  wMeas/1 -> Add/2
  Discrete-Time Integrator/1 -> Add1/2
  Kp/1 -> Add1/1
  wRef/1 -> Add/1

== system ssc_auto_ev_20b/Step 2: Multirate Model/Battery/Electric and Thermal Model/Thermal Model ==
  Battery Thermal Mass : fl_lib/Thermal/Thermal Elements/Thermal Mass  Commented=on  mass=cell_mass*Nseries*Nparallel kg  sp_heat=cell_Cp_heat J/kg/K  T_specify=on  T_priority=High  T=T_init K  T_nominal_specify=off  T_nominal_unit=K  T_nominal_value=1  Q_specify=off  Q_priority=High  Q=0 J/s  Q_nominal_specify=off  Q_nominal_unit=J/s  Q_nominal_value=1
      settings: SourceProductBaseCode=PW,SS,VE
  Heat Flow Source : fl_lib/Thermal/Thermal Sources/Controlled Heat Flow Rate Source
      settings: SourceProductBaseCode=PW,SS,VE
  Ideal Temperature Sensor : fl_lib/Thermal/Thermal Sensors/Temperature Sensor
      settings: SourceProductBaseCode=PW,SS,VE
  ThRef1 : fl_lib/Thermal/Thermal Elements/Thermal Reference
      settings: SourceProductBaseCode=PW,SS,VE
  ThRef2 : fl_lib/Thermal/Thermal Elements/Thermal Reference
      settings: SourceProductBaseCode=PW,SS,VE
  PlossTotal : PMIOPort  Tag=PMCPort  Side=Left
  T : PMIOPort  Tag=PMCPort  Port=2  Side=Right
  H : PMIOPort  Tag=PMCPort  Port=3  Side=Left
  connections:
  Heat Flow Source/RConn1 -- PlossTotal/RConn1
  Heat Flow Source/LConn1 -- Battery Thermal Mass/LConn1 -- H/RConn1 -- Ideal Temperature Sensor/LConn1
  ThRef1/LConn1 -- Heat Flow Source/RConn2
  Ideal Temperature Sensor/RConn2 -- T/RConn1
  ThRef2/LConn1 -- Ideal Temperature Sensor/RConn1

== system ssc_auto_ev_20b/Step 2: Multirate Model/Battery Thermal Mass/Port 1 Interface/Interface ==
  through1 : Inport
  through2 : Inport  Port=2
  Continuous : Subsystem  VariantControl=Continuous
  Discrete : Subsystem  VariantControl=Discrete
  across2 : Outport
  across1 : Outport  Port=2

== system ssc_auto_ev_20b/Step 2: Multirate Model/Cooling System/ Heat Exchanger Characteristic/Characteristic ==
  PS Product : fl_lib/Physical Signals/Functions/PS Product
      settings: SourceProductBaseCode=PW,SS,VE
  PS Subtract : fl_lib/Physical Signals/Functions/PS Subtract
      settings: SourceProductBaseCode=PW,SS,VE
  Specific dissipation (J/s/K) per unit mass flow rate : fl_lib/Physical Signals/Functions/PS Gain  gain=100 J/s/(kg/s)/K
      settings: SourceProductBaseCode=PW,SS,VE
  M : PMIOPort  Side=Right
  T in : PMIOPort  Port=2  Side=Right
  T Env : PMIOPort  Port=3  Side=Right
  Q : PMIOPort  Port=4  Side=Left
  connections:
  PS Product/LConn2 -- Specific dissipation (J/s/K) per unit mass flow rate/RConn1
  Specific dissipation (J/s/K) per unit mass flow rate/LConn1 -- M/RConn1
  PS Subtract/LConn2 -- T in/RConn1
  PS Subtract/RConn1 -- PS Product/LConn1
  PS Product/RConn1 -- Q/RConn1
  PS Subtract/LConn1 -- T Env/RConn1

== system ssc_auto_ev_20b/Step 2: Multirate Model/Cooling System/Heat Exchanger Characteristic/Characteristic ==
  PS Product1 : fl_lib/Physical Signals/Functions/PS Product
      settings: SourceProductBaseCode=PW,SS,VE
  PS Subtract : fl_lib/Physical Signals/Functions/PS Subtract
      settings: SourceProductBaseCode=PW,SS,VE
  Specific dissipation : fl_lib/Physical Signals/Lookup Tables/PS Lookup Table (1D)  x="[0 0.2 0.4  0.7  1 1.2  1.4  2.5 ] kg/s"  f=10000 * [0 0.5 0.75 0.92 1 1.02 1.03 1.04] J/s/K  interp_method=simscape.enum.interpolation.linear  extrap_method=simscape.enum.extrapolation.linear
      settings: SourceProductBaseCode=PW,SS,VE
  Mass Flow : PMIOPort  Side=Left
  Temp Inlet : PMIOPort  Port=2  Side=Left
  Temp Motor : PMIOPort  Port=3  Side=Left
  Q : PMIOPort  Port=4  Side=Right
  connections:
  Specific dissipation/LConn1 -- Mass Flow/RConn1
  Q/RConn1 -- PS Product1/RConn1
  PS Subtract/LConn2 -- Temp Inlet/RConn1
  PS Subtract/LConn1 -- Temp Motor/RConn1
  PS Product1/LConn2 -- Specific dissipation/RConn1
  PS Product1/LConn1 -- PS Subtract/RConn1

== system ssc_auto_ev_20b/Step 2: Multirate Model/Network Coupler (Flexible Shaft)/Port 1 Interface/Interface ==
  across1 : Inport
  across2 : Inport  Port=2
  Continuous : Subsystem  VariantControl=Continuous
  Discrete : Subsystem  VariantControl=Discrete
  through2 : Outport
  through1 : Outport  Port=2

== system ssc_auto_ev_20b/Step 2: Multirate Model/Network Coupler (Voltage-Current)/Port 1 Interface/Interface ==
  through1 : Inport
  across2 : Inport  Port=2
  Continuous : Subsystem  VariantControl=Continuous
  Discrete : Subsystem  VariantControl=Discrete
  through2 : Outport
  across1 : Outport  Port=2

== system ssc_auto_ev_20b/Step 2: Multirate Model/Rotor Iron Thermal Mass//1/Port 1 Interface/Interface ==
  through1 : Inport
  through2 : Inport  Port=2
  Continuous : Subsystem  VariantControl=Continuous
  Discrete : Subsystem  VariantControl=Discrete
  across2 : Outport
  across1 : Outport  Port=2

== system ssc_auto_ev_20b/Step 2: Multirate Model/Rotor Iron Thermal Mass//2/Port 1 Interface/Interface ==
  through1 : Inport
  through2 : Inport  Port=2
  Continuous : Subsystem  VariantControl=Continuous
  Discrete : Subsystem  VariantControl=Discrete
  across2 : Outport
  across1 : Outport  Port=2

== system ssc_auto_ev_20b/Step 2: Multirate Model/Vehicle Dynamics/Brake Torque/Smooth Sign ==
  1 : fl_lib/Physical Signals/Sources/PS Constant  constant=1
      settings: SourceProductBaseCode=PW,SS,VE
  2 : fl_lib/Physical Signals/Functions/PS Gain  gain=2 1/(rad/s)
      settings: SourceProductBaseCode=PW,SS,VE
  PS Add : fl_lib/Physical Signals/Functions/PS Add
      settings: SourceProductBaseCode=PW,SS,VE
  PS Subtract : fl_lib/Physical Signals/Functions/PS Subtract
      settings: SourceProductBaseCode=PW,SS,VE
  exp(2x) : fl_lib/Physical Signals/Functions/PS Math Function  fcn_choice=foundation.enum.math_function.exp
      settings: SourceProductBaseCode=PW,SS,VE
  tanh(x) : fl_lib/Physical Signals/Functions/PS Divide
      settings: SourceProductBaseCode=PW,SS,VE
  x : PMIOPort  Side=Left
  y : PMIOPort  Port=2  Side=Right
  connections:
  1/RConn1 -- PS Subtract/LConn2 -- PS Add/LConn1
  exp(2x)/LConn1 -- 2/RConn1
  exp(2x)/RConn1 -- PS Subtract/LConn1 -- PS Add/LConn2
  tanh(x)/LConn2 -- PS Add/RConn1
  tanh(x)/LConn1 -- PS Subtract/RConn1
  2/LConn1 -- x/RConn1
  tanh(x)/RConn1 -- y/RConn1

== system ssc_auto_ev_20b/Step 2: Multirate Model/Vehicle Control/Cruise Control/Capture speed ==
  In1 : Inport
  Trigger : TriggerPort  VariantControl=Variant
  Out1 : Outport  VectorParamsAs1DForOutWhenUnconnected=off
  wires:
  In1/1 -> Out1/1

== system ssc_auto_ev_20b/Step 2: Multirate Model/Vehicle Control/Cruise Control/Speed Controller ==
  wRef : Inport
  wMeas : Inport  Port=2
  Add : Sum  Inputs=|+-
  Add1 : Sum
  Discrete-Time Integrator : DiscreteIntegrator  gainval=Ki  SampleTime=ts  LimitOutput=on  UpperSaturationLimit=trqMax  LowerSaturationLimit=-trqMax  ICPrevOutput=DiscIntNeverNeededParam  ICPrevScaledInput=DiscIntNeverNeededParam
  Kp : Gain  Gain=Kp
  trqRef : Outport  VectorParamsAs1DForOutWhenUnconnected=off
  wires:
  Add/1 -> Discrete-Time Integrator/1, Kp/1
  Add1/1 -> trqRef/1
  wMeas/1 -> Add/2
  Discrete-Time Integrator/1 -> Add1/2
  Kp/1 -> Add1/1
  wRef/1 -> Add/1

== system ssc_auto_ev_20b/Step 3: Ungroup and Redraw/Battery/Electric and Thermal Model/Thermal Model ==
  Battery Thermal Mass : fl_lib/Thermal/Thermal Elements/Thermal Mass  Commented=on  mass=cell_mass*Nseries*Nparallel kg  sp_heat=cell_Cp_heat J/kg/K  T_specify=on  T_priority=High  T=T_init K  T_nominal_specify=off  T_nominal_unit=K  T_nominal_value=1  Q_specify=off  Q_priority=High  Q=0 J/s  Q_nominal_specify=off  Q_nominal_unit=J/s  Q_nominal_value=1
      settings: SourceProductBaseCode=PW,SS,VE
  Heat Flow Source : fl_lib/Thermal/Thermal Sources/Controlled Heat Flow Rate Source
      settings: SourceProductBaseCode=PW,SS,VE
  Ideal Temperature Sensor : fl_lib/Thermal/Thermal Sensors/Temperature Sensor
      settings: SourceProductBaseCode=PW,SS,VE
  ThRef1 : fl_lib/Thermal/Thermal Elements/Thermal Reference
      settings: SourceProductBaseCode=PW,SS,VE
  ThRef2 : fl_lib/Thermal/Thermal Elements/Thermal Reference
      settings: SourceProductBaseCode=PW,SS,VE
  PlossTotal : PMIOPort  Tag=PMCPort  Side=Left
  T : PMIOPort  Tag=PMCPort  Port=2  Side=Right
  H : PMIOPort  Tag=PMCPort  Port=3  Side=Left
  connections:
  ThRef2/LConn1 -- Ideal Temperature Sensor/RConn1
  Ideal Temperature Sensor/RConn2 -- T/RConn1
  ThRef1/LConn1 -- Heat Flow Source/RConn2
  Ideal Temperature Sensor/LConn1 -- H/RConn1 -- Battery Thermal Mass/LConn1 -- Heat Flow Source/LConn1
  Heat Flow Source/RConn1 -- PlossTotal/RConn1

== system ssc_auto_ev_20b/Step 3: Ungroup and Redraw/Cooling System/ Heat Exchanger Characteristic/Characteristic ==
  PS Product : fl_lib/Physical Signals/Functions/PS Product
      settings: SourceProductBaseCode=PW,SS,VE
  PS Subtract : fl_lib/Physical Signals/Functions/PS Subtract
      settings: SourceProductBaseCode=PW,SS,VE
  Specific dissipation (J/s/K) per unit mass flow rate : fl_lib/Physical Signals/Functions/PS Gain  gain=100 J/s/(kg/s)/K
      settings: SourceProductBaseCode=PW,SS,VE
  M : PMIOPort  Side=Right
  T in : PMIOPort  Port=2  Side=Right
  T Env : PMIOPort  Port=3  Side=Right
  Q : PMIOPort  Port=4  Side=Left
  connections:
  PS Subtract/LConn1 -- T Env/RConn1
  PS Product/RConn1 -- Q/RConn1
  PS Subtract/RConn1 -- PS Product/LConn1
  PS Subtract/LConn2 -- T in/RConn1
  Specific dissipation (J/s/K) per unit mass flow rate/LConn1 -- M/RConn1
  PS Product/LConn2 -- Specific dissipation (J/s/K) per unit mass flow rate/RConn1

== system ssc_auto_ev_20b/Step 3: Ungroup and Redraw/Cooling System/Heat Exchanger Characteristic/Characteristic ==
  PS Product1 : fl_lib/Physical Signals/Functions/PS Product
      settings: SourceProductBaseCode=PW,SS,VE
  PS Subtract : fl_lib/Physical Signals/Functions/PS Subtract
      settings: SourceProductBaseCode=PW,SS,VE
  Specific dissipation : fl_lib/Physical Signals/Lookup Tables/PS Lookup Table (1D)  x="[0 0.2 0.4  0.7  1 1.2  1.4  2.5 ] kg/s"  f=10000 * [0 0.5 0.75 0.92 1 1.02 1.03 1.04] J/s/K  interp_method=simscape.enum.interpolation.linear  extrap_method=simscape.enum.extrapolation.linear
      settings: SourceProductBaseCode=PW,SS,VE
  Mass Flow : PMIOPort  Side=Left
  Temp Inlet : PMIOPort  Port=2  Side=Left
  Temp Motor : PMIOPort  Port=3  Side=Left
  Q : PMIOPort  Port=4  Side=Right
  connections:
  PS Product1/LConn1 -- PS Subtract/RConn1
  PS Product1/LConn2 -- Specific dissipation/RConn1
  PS Subtract/LConn1 -- Temp Motor/RConn1
  PS Subtract/LConn2 -- Temp Inlet/RConn1
  Q/RConn1 -- PS Product1/RConn1
  Specific dissipation/LConn1 -- Mass Flow/RConn1

== system ssc_auto_ev_20b/Step 3: Ungroup and Redraw/Port 1 Interface/Interface/Continuous ==
  through2 : Inport
  through1 : Inport  Port=2
  1/thermalMass : Gain  Gain=1/thermalMass  SaturateOnIntegerOverflow=on  OutDataTypeStr=Inherit: Same as input  ParamDataTypeStr=Inherit: Same as input
  Integrator : Integrator  InitialCondition=T0
  Prediction : Subsystem  Commented=through  mask(Prediction (discrete->continuous)){h2=h2}
      mask prompts: h2 "physmod:simscape:couplers:SimscapeNetworkCouplersLib:PortUDiscreteSampleTimes_MP"
      mask help: physmod:simscape:couplers:SimscapeNetworkCouplersLib:Predictiondiscretecontinuous_MD
  Smoothing : Subsystem  Commented=through  mask(Smoothing (continuous->discrete)){tsSmoothing=tsSmoothing, smoothing0=T0}
      mask prompts: tsSmoothing "physmod:simscape:couplers:SimscapeNetworkCouplersLib:SmoothingTimeConstants_MP"; smoothing0 "physmod:simscape:couplers:SimscapeNetworkCouplersLib:InitialOutput_MP"
      mask help: physmod:simscape:couplers:SimscapeNetworkCouplersLib:Smoothingcontinuousdiscrete_MD
  Sum : Sum  InputSameDT=on  SaturateOnIntegerOverflow=on  OutDataTypeStr=Inherit: Same as first input
  across2 : Outport
  across1 : Outport  Port=2
  wires:
  Integrator/1 -> Smoothing/1(u), across1/1
  1/thermalMass/1 -> Integrator/1
  Sum/1 -> 1/thermalMass/1
  Smoothing/1(y) -> across2/1
  Prediction/1(y) -> Sum/2
  through1/1 -> Sum/1
  through2/1 -> Prediction/1(u)

== system ssc_auto_ev_20b/Step 3: Ungroup and Redraw/Port 1 Interface/Interface/Discrete ==
  through2 : Inport
  through1 : Inport  Port=2
  1/thermalMass : Gain  Gain=1/thermalMass  SaturateOnIntegerOverflow=on  OutDataTypeStr=Inherit: Same as input  ParamDataTypeStr=Inherit: Same as input
  Integrator : DiscreteIntegrator  InitialCondition=T0  SampleTime=h1  ICPrevOutput=DiscIntNeverNeededParam  ICPrevScaledInput=DiscIntNeverNeededParam
  Prediction : Subsystem  Commented=through  mask(Prediction (slow->fast)){h2=h2, h1=h1}
      mask prompts: h2 "physmod:simscape:couplers:SimscapeNetworkCouplersLib:PortUDiscreteSampleTimes_MP"; h1 "physmod:simscape:couplers:SimscapeNetworkCouplersLib:PortYDiscreteSampleTimes_MP"
      mask help: physmod:simscape:couplers:SimscapeNetworkCouplersLib:Predictionslowfast_MD
  Smoothing : Subsystem  Commented=through  mask(Smoothing (fast->slow)){nSmooth=nSmooth, h1=h1, smoothing0=T0}
      mask prompts: nSmooth "physmod:simscape:couplers:SimscapeNetworkCouplersLib:NumberOfSamplesOverWhichToSmooth_MP"; h1 "physmod:simscape:couplers:SimscapeNetworkCouplersLib:PortUDiscreteSampleTimes_MP"; smoothing0 "physmod:simscape:couplers:SimscapeNetworkCouplersLib:InitialOutput_MP"
      mask help: physmod:simscape:couplers:SimscapeNetworkCouplersLib:Smoothingfastslow_MD
  Sum : Sum  InputSameDT=on  SaturateOnIntegerOverflow=on  OutDataTypeStr=Inherit: Same as first input
  across2 : Outport
  across1 : Outport  Port=2
  wires:
  1/thermalMass/1 -> Integrator/1
  Sum/1 -> 1/thermalMass/1
  Integrator/1 -> Smoothing/1(u), across1/1
  Smoothing/1(y) -> across2/1
  Prediction/1(y) -> Sum/2
  through2/1 -> Prediction/1(u)
  through1/1 -> Sum/1
